simulink model "lcd_project"  (R2016a)
settings: Solver=FixedStepAuto  StartTime=0.0  StopTime=inf  RelTol=1e-3
libraries: arduinolib x1
settings Model: SimulationMode=external  ExtModeTrigDuration=2  Creator=mmdclm  LastModifiedBy=Lara
settings OptimizationCC: OptimizeModelRefInitCode=on  LifeSpan=1  MaxStackSize=64
settings HardwareCC: ProdBitPerInt=16  ProdBitPerPointer=16  ProdLargestAtomicFloat=None  ProdWordSize=8  ProdHWDeviceType=Atmel->AVR
settings RTWCC: SystemTargetFile=ert.tlc  HardwareBoard=Arduino Uno  TemplateMakefile=ert_default_tmf  GenerateReport=on  Toolchain=Arduino AVR v1.6.1  BuildConfiguration=Faster Runs  IncludeHyperlinkInReport=on  LaunchReport=on  GenerateTraceInfo=on  GenerateTraceReport=on  GenerateTraceReportSl=on  GenerateTraceReportSf=on  GenerateTraceReportEml=on
settings CodeAppCC: ForceParamTrailComments=on  IgnoreCustomStorageClasses=off  OperatorAnnotations=on  SimulinkDataObjDesc=on  SFDataObjDesc=on  MATLABFcnDesc=on  InsertBlockDesc=on  MATLABSourceComments=on
settings ERTTargetCC: SupportContinuousTime=on  SupportNonInlinedSFcns=on  SupportVariableSizeSignals=on

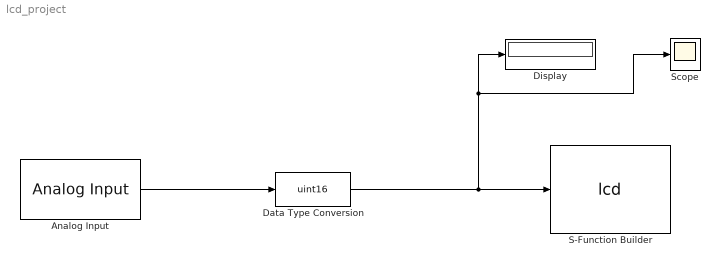
== system lcd_project ==
  Analog Input : arduinolib/Analog Input  pinNumber=0  sampleTime=0.01  blockPlatform=arduino
  Data Type Conversion : DataTypeConversion  OutDataTypeStr=uint16
  Display : Display
  S-Function Builder : S-Function  InitFcn=try, set_param(gcb,'FunctionName','lcd'), end  FunctionName=lcd  SFunctionModules=lcd_wrapper  SFunctionDeploymentMode=off  EnableBusSupport=off  mask(S-Function Builder){}
      mask help: Simulink:masks:SFunctionBuilder_MD
      mask init:
      | val = [[.9  0.75 0.75 1 1 .9 .9 1]',[1 1 0.75 0.75 .9 .9 1 .9]'];try , sys = get_param(gcb,'SfunBuilderFcnName');if isempty(sys), sys = get_param(gcb,'FunctionName'); end,catch, sys = get_param(gcb,'FunctionName'); end
      settings: CopyFcn=set_param(gcbh,'LinkStatus','none')  PreSaveFcn=try, set_param(gcb,'FunctionName','lcd'), end  OpenFcn=sfunctionwizard(gcbh)
      mask Display: plot(val(:,1),val(:,2)),disp(sys), port_label('input',1,'Char_val')
  Scope : Scope
  wires:
  Analog Input/1 -> Data Type Conversion/1
  Data Type Conversion/1 -> Scope/1, Display/1, S-Function Builder/1
